simulink model "cbf_HO_with_lead_accel"  (R2023b)
settings: Solver=FixedStepAuto  StartTime=0.0  StopTime=inf  FixedStep=0.05  RelTol=1e-3
undefined symbols (not defined in the file): Angular, Linear
libraries: robotlib x16
settings Model: Creator=ivory  LastModifiedBy=vanderbilt
settings SolverCC: AlgebraicLoopSolver=TrustRegion
settings OptimizationCC: EnhancedBackFolding=on  PassReuseOutputArgsAs=Individual arguments  ZeroExternalMemoryAtStartup=off  ZeroInternalMemoryAtStartup=off  MaxStackSize=64  OptimizeBlockOrder=speed  DifferentSizesBufferReuse=on  OptimizationCustomize=off  EfficientTunableParamExpr=on
settings DebuggingCC: ParameterTunabilityLossMsg=error  UnconnectedInputMsg=warning  UnconnectedOutputMsg=warning  UnconnectedLineMsg=warning
settings HardwareCC: ProdBitPerPointer=32  ProdBitPerSizeT=32  ProdBitPerPtrDiffT=32  ProdLargestAtomicFloat=None  ProdIntDivRoundTo=Undefined  ProdEndianess=Unspecified  ProdWordSize=32  ProdHWDeviceType=Generic->Unspecified (assume 32-bit Generic)
settings ModelReferenceCC: EnableRefExpFcnMdlSchedulingChecks=on
settings SFSimCC: MATLABDynamicMemAlloc=off  SimTargetLang=C++
settings RTWCC: Description=Embedded Coder  SystemTargetFile=ert.tlc  HardwareBoard=Robot Operating System (ROS)  TLCOptions="-aInlineSetEventsForThisBaseRateFcn=TLC_FALSE -aSuppressMultiTaskScheduler=TLC_FALSE  -aRateBasedStepFcn=0"  GenCodeOnly=on  TemplateMakefile=ert_default_tmf  GenerateReport=on  Toolchain=Catkin  IncludeHyperlinkInReport=on  LaunchReport=on  TargetLang=C++  GenerateTraceInfo=on  GenerateTraceReport=on  GenerateTraceReportSl=on  GenerateTraceReportSf=on  GenerateTraceReportEml=on  DLArmComputeVersion=19.05
settings CodeAppCC: ForceParamTrailComments=on  IgnoreCustomStorageClasses=off  OperatorAnnotations=on  SimulinkDataObjDesc=on  SFDataObjDesc=on  InsertBlockDesc=on
settings ERTTargetCC: SupportContinuousTime=on  SupportVariableSizeSignals=on

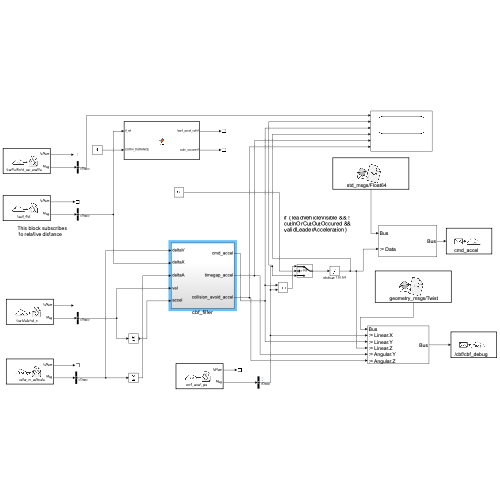
[thumbnail: Simulink's stored preview of the top-level diagram]
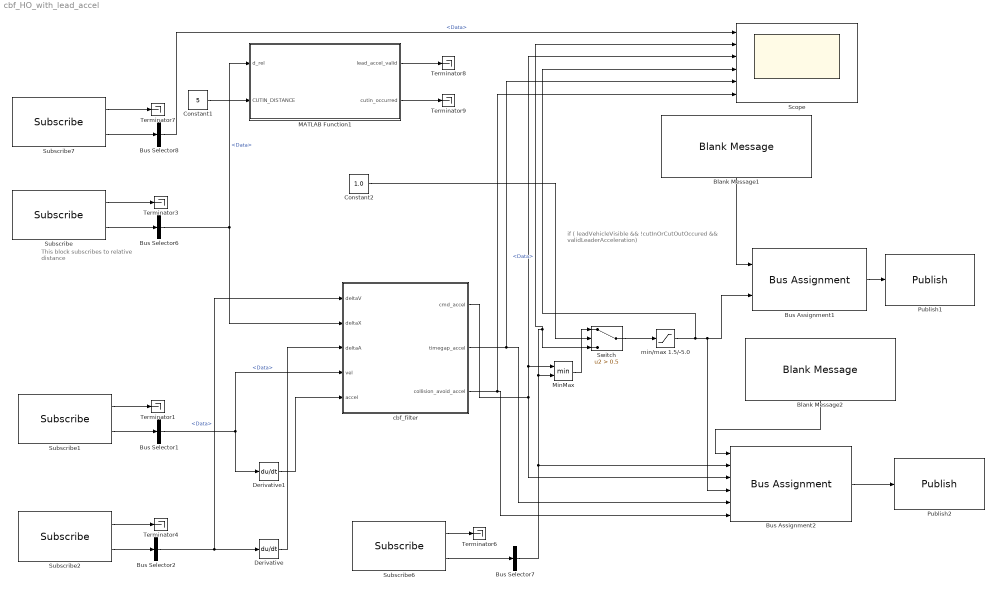
== system cbf_HO_with_lead_accel ==
  note: if ( leadVehicleVisible && !cutInOrCutOutOccured && validLeaderAcceleration)
  note: This block subscribes
      | to relative distance
  Blank Message1 : robotlib/Blank Message  messageClass=Message  entityType=std_msgs/Float64  messageType=std_msgs/Float64  SampleTime=inf  legacyBusStruct=off
  Blank Message2 : robotlib/Blank Message  messageClass=Message  entityType=geometry_msgs/Twist  messageType=geometry_msgs/Twist  SampleTime=inf  legacyBusStruct=off
  Bus Assignment1 : BusAssignment  AssignedSignals=Data
  Bus Assignment2 : BusAssignment  AssignedSignals=Linear.X,Linear.Y,Linear.Z,Angular.Y,Angular.Z
  Bus Selector{1..2,6..8} (5 alike) : BusSelector  OutputSignals=Data
  Constant1 : Constant  Value=5
  Constant2 : Constant  Value=1.0
  Derivative : Derivative
  Derivative1 : Derivative
  MATLAB Function1 : MATLAB Function  TreatAsAtomicUnit=on
  MinMax : MinMax  Inputs=2
  Publish1 : robotlib/Publish  topicSource=Specify your own  topic=cmd_accel  messageType=std_msgs/Float64  legacyBusStruct=off  messageQueueLength=1
  Publish2 : robotlib/Publish  topicSource=Specify your own  topic=/cbf/cbf_debug  messageType=geometry_msgs/Twist  legacyBusStruct=off  messageQueueLength=1
  Scope : Scope  NumInputPorts=6
  Subscribe : robotlib/Subscribe  topicSource=Specify your own  topic=lead_dist  messageType=std_msgs/Float64  SampleTime=-1  legacyBusStruct=off  messageQueueLength=1
  Subscribe1 : robotlib/Subscribe  topicSource=Specify your own  topic=/car/state/vel_x  messageType=std_msgs/Float64  SampleTime=-1  legacyBusStruct=off  messageQueueLength=1
  Subscribe2 : robotlib/Subscribe  topicSource=Specify your own  topic=radar_rv_estimate  messageType=std_msgs/Float64  SampleTime=-1  legacyBusStruct=off  messageQueueLength=1
  Subscribe6 : robotlib/Subscribe  topicSource=Specify your own  topic=cmd_accel_pre  messageType=std_msgs/Float64  SampleTime=-1  legacyBusStruct=off  messageQueueLength=1
  Subscribe7 : robotlib/Subscribe  topicSource=Specify your own  topic=/car/hud/mini_car_enable  messageType=std_msgs/Bool  SampleTime=-1  legacyBusStruct=off  messageQueueLength=1
  Switch : Switch  Criteria=u2 > Threshold  Threshold=0.5  SaturateOnIntegerOverflow=off  InputSameDT=off
  Terminator{1,3..4,6..9} (7 alike) : Terminator
  cbf_filter : Subsystem
  min/max 1.5/-5.0 : Saturate  UpperLimit=1.5  LowerLimit=-5.0
  wires:
  MATLAB Function1/1(lead_accel_valid) -> Terminator8/1
  MinMax/1 -> Switch/1
  Bus Selector8/1 -> Scope/1  "<Data>"
  Subscribe7/2 -> Bus Selector8/1
  Subscribe2/1 -> Terminator4/1
  Subscribe1/1 -> Terminator1/1
  Bus Assignment1/1 -> Publish1/1
  Bus Selector7/1 -> Bus Assignment2/2, MinMax/2, Switch/3, Scope/2  "<Data>"
  Subscribe2/2 -> Bus Selector2/1
  cbf_filter/1(cmd_accel) -> Scope/3, MinMax/1, Bus Assignment2/3
  Bus Selector6/1 -> MATLAB Function1/1(d_rel), cbf_filter/2(deltaX)  "<Data>"
  Bus Assignment2/1 -> Publish2/1
  Subscribe7/1 -> Terminator7/1
  Subscribe/1 -> Terminator3/1
  cbf_filter/3(collision_avoid_accel) -> Scope/6, Bus Assignment2/6
  Constant1/1 -> MATLAB Function1/2(CUTIN_DISTANCE)
  Switch/1 -> min/max 1.5/-5.0/1
  Bus Selector2/1 -> Derivative/1, cbf_filter/1(deltaV)  "<Data>"
  Subscribe6/1 -> Terminator6/1
  Blank Message1/1 -> Bus Assignment1/1
  min/max 1.5/-5.0/1 -> Scope/4, Bus Assignment2/4, Bus Assignment1/2
  Subscribe1/2 -> Bus Selector1/1
  MATLAB Function1/2(cutin_occurred) -> Terminator9/1
  cbf_filter/2(timegap_accel) -> Scope/5, Bus Assignment2/5
  Bus Selector1/1 -> Derivative1/1, cbf_filter/4(vel)  "<Data>"
  Subscribe/2 -> Bus Selector6/1
  Constant2/1 -> Switch/2
  Blank Message2/1 -> Bus Assignment2/1
  Subscribe6/2 -> Bus Selector7/1
  Derivative/1 -> cbf_filter/3(deltaA)
  Derivative1/1 -> cbf_filter/5(accel)

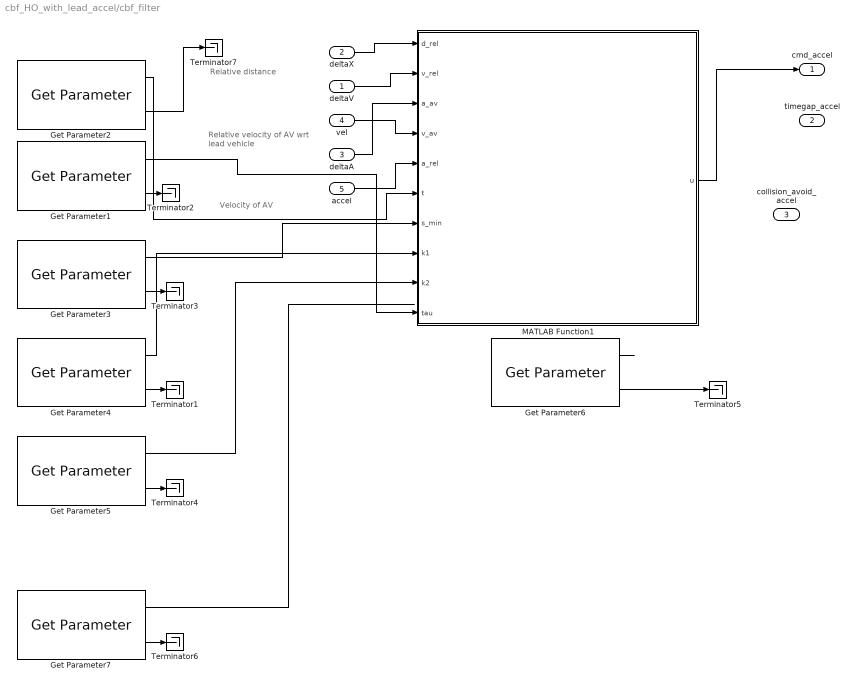
== system cbf_HO_with_lead_accel/cbf_filter ==
  note: Velocity of AV
  note: Relative velocity of
      | AV wrt lead vehicle
  note: Relative distance
  deltaV : Inport
  deltaX : Inport  Port=2
  deltaA : Inport  Port=3
  vel : Inport  Port=4
  accel : Inport  Port=5
  Get Parameter1 : robotlib/Get Parameter  ParameterSource=Specify your own  ParameterName=k_timegap  ParameterType=double  ParameterMaxArrayLength=16  ParameterInitialValue=0.1  SampleTime=-1  ShowErrorCodeOutput=on  ModelName=cbf_HO_with_lead_accel  BlockId=ParamGet_cbf_HO_with_lead_accel_566
  Get Parameter2 : robotlib/Get Parameter  ParameterSource=Specify your own  ParameterName=timegap  ParameterType=double  ParameterMaxArrayLength=16  ParameterInitialValue=2.0  SampleTime=-1  ShowErrorCodeOutput=on  ModelName=cbf_HO_with_lead_accel  BlockId=ParamGet_cbf_HO_with_lead_accel_567
  Get Parameter3 : robotlib/Get Parameter  ParameterSource=Specify your own  ParameterName=s_min  ParameterType=double  ParameterMaxArrayLength=16  ParameterInitialValue=15.0  SampleTime=-1  ShowErrorCodeOutput=on  ModelName=cbf_HO_with_lead_accel  BlockId=ParamGet_cbf_HO_with_lead_accel_568
  Get Parameter4 : robotlib/Get Parameter  ParameterSource=Specify your own  ParameterName=k1  ParameterType=double  ParameterMaxArrayLength=16  ParameterInitialValue=0.5  SampleTime=-1  ShowErrorCodeOutput=on  ModelName=cbf_HO_with_lead_accel  BlockId=ParamGet_cbf_HO_with_lead_accel_569
  Get Parameter5 : robotlib/Get Parameter  ParameterSource=Specify your own  ParameterName=k2  ParameterType=double  ParameterMaxArrayLength=16  ParameterInitialValue=0.5  SampleTime=-1  ShowErrorCodeOutput=on  ModelName=cbf_HO_with_lead_accel  BlockId=ParamGet_cbf_HO_with_lead_accel_570
  Get Parameter6 : robotlib/Get Parameter  ParameterSource=Specify your own  ParameterName=w3  ParameterType=double  ParameterMaxArrayLength=16  ParameterInitialValue=6.0  SampleTime=-1  ShowErrorCodeOutput=on  ModelName=cbf_HO_with_lead_accel  BlockId=ParamGet_cbf_HO_with_lead_accel_571
  Get Parameter7 : robotlib/Get Parameter  ParameterSource=Specify your own  ParameterName=tau  ParameterType=double  ParameterMaxArrayLength=16  ParameterInitialValue=1.5  SampleTime=-1  ShowErrorCodeOutput=on  ModelName=cbf_HO_with_lead_accel  BlockId=ParamGet_cbf_HO_with_lead_accel_595
  MATLAB Function1 : MATLAB Function  TreatAsAtomicUnit=on
  Terminator{1..7} (7 alike) : Terminator
  cmd_accel : Outport
  timegap_accel : Outport  Port=2
  collision_avoid_accel : Outport  Port=3
  wires:
  Get Parameter4/1 -> MATLAB Function1/8(k1)
  Get Parameter4/2 -> Terminator1/1
  Get Parameter2/1 -> MATLAB Function1/6(t)
  Get Parameter2/2 -> Terminator7/1
  Get Parameter3/2 -> Terminator3/1
  Get Parameter1/1 -> MATLAB Function1/10(tau)
  Get Parameter1/2 -> Terminator2/1
  Get Parameter3/1 -> MATLAB Function1/7(s_min)
  ? -> timegap_accel/1
  MATLAB Function1/1(u) -> cmd_accel/1
  vel/1 -> MATLAB Function1/4(v_av)
  deltaV/1 -> MATLAB Function1/2(v_rel)
  deltaX/1 -> MATLAB Function1/1(d_rel)
  Get Parameter5/2 -> Terminator4/1
  Get Parameter5/1 -> MATLAB Function1/9(k2)
  Get Parameter6/1 -> ?
  Get Parameter6/2 -> Terminator5/1
  ? -> collision_avoid_accel/1
  deltaA/1 -> MATLAB Function1/3(a_av)
  accel/1 -> MATLAB Function1/5(a_rel)
  Get Parameter7/2 -> Terminator6/1
  Get Parameter7/1 -> ?

== matlab function cbf_HO_with_lead_accel/cbf_filter/MATLAB Function1 ==
  data: u output; d_rel input; v_rel input; a_av input; v_av input; a_rel input; t input; s_min input; k1 input; k2 input; tau input
function u = fcn(d_rel,v_rel,a_av, v_av, a_rel, t,s_min,k1,k2,tau)
%% calculates cbf acceleration given a model with first-order lag on accel:

h = (d_rel - t*v_av - s_min);

dh_dt = (v_rel - t*a_av);

u = (tau/t)*(a_rel + (t/tau)*a_av + (k1+k2)*(dh_dt) + (k1*k2)*h);

== matlab function cbf_HO_with_lead_accel/MATLAB Function1 ==
  data: lead_accel_valid output; d_rel input; CUTIN_DISTANCE input; cutin_occurred output
function [lead_accel_valid, cutin_occurred]= fcn(d_rel,CUTIN_DISTANCE)
%#codegen

persistent relative_distance_prev;
if isempty(relative_distance_prev)
    relative_distance_prev=d_rel;
end

cutin_occurred = 1;
lead_accel_valid=1;

if( abs( relative_distance_prev - d_rel ) > CUTIN_DISTANCE )
    cutin_occurred = 1;
else
    cutin_occurred = 0;
end

relative_distance_prev = d_rel;
